simulink model "slow"  (R2019b)
settings: Solver=FixedStepDiscrete  StartTime=0.0  StopTime=25  FixedStep=Ts_ctrl  RelTol=1e-3
model workspace: external: MAT-File (data not in the file)
values from neighbouring files (symbols this model uses):
  CCR_max = 5250    [datasheet.m]
  delay_input = 0    [codegen_init.m]
  dpole_cut = exp(-w_cut*Ts_ctrl)    [codegen_init.m]
  encoder_res = 4096    [datasheet.m]
  g = 9.81    [datasheet.m]
  Jp = Jp_cm + mp*lp^2    (= 0.004290672)    [datasheet.m]
  Larm = 0.216    [datasheet.m]
  lp = 0.156    [datasheet.m]
  mp = 0.127    [datasheet.m]
  par_ctrl = Simulink.Parameter(par_ctrl)    [codegen_init.m]
  par_dn = Simulink.Parameter(par_dn)    [codegen_init.m]
  th_lim = 30/180*pi    (= 0.523598775598)    [codegen_init.m]
  Ts_ctrl = 5e-3    (= 0.005)    [codegen_init.m]
  volt_max = 6    [datasheet.m]
undefined symbols (not defined in the file or in its folder): state_board_init, state_pc_init
settings Model: OrderedModelArguments=off  Creator=Simone  LastModifiedBy=simone
settings OptimizationCC: DefaultParameterBehavior=Inlined  GainParamInheritBuiltInType=on  UseFloatMulNetSlope=on  UseSpecifiedMinMax=on  InlineInvariantSignals=on  PassReuseOutputArgsAs=Individual arguments  ZeroExternalMemoryAtStartup=off  ZeroInternalMemoryAtStartup=off  NoFixptDivByZeroProtection=on  EfficientFloat2IntCast=on  LifeSpan=1  OptimizeBlockOrder=speed  EfficientTunableParamExpr=on
settings DebuggingCC: SignalInfNanChecking=error  ParameterPrecisionLossMsg=error  ParameterTunabilityLossMsg=error
settings HardwareCC: ProdBitPerLong=64  ProdLongLongMode=on  ProdHWDeviceType=Intel->x86-64 (Linux 64)
settings SFSimCC: MATLABDynamicMemAlloc=off
settings RTWCC: SystemTargetFile=ert.tlc  GenCodeOnly=on  PackageGeneratedCodeAndArtifacts=on  TemplateMakefile=ert_default_tmf  GenerateReport=on  Toolchain=GNU gcc/g++ | gmake (64-bit Linux)  BuildConfiguration=Faster Runs  IncludeHyperlinkInReport=on  LaunchReport=on  GenerateTraceInfo=on  GenerateTraceReport=on  GenerateTraceReportSl=on  GenerateTraceReportSf=on  GenerateTraceReportEml=on  CheckMdlBeforeBuild=Error
settings CodeAppCC: ForceParamTrailComments=on  IgnoreCustomStorageClasses=off  OperatorAnnotations=on  SimulinkDataObjDesc=on  SFDataObjDesc=on  MATLABFcnDesc=on  InsertBlockDesc=on  StateflowObjectComments=on  MATLABSourceComments=on  EnableCustomComments=on  ReqsInCode=on
settings ERTTargetCC: TargetLangStandard=C99 (ISO)  UtilityFuncGeneration=Shared location  CombineSignalStateStructs=on  SuppressErrorStatus=on  SupportAbsoluteTime=off  SupportNonFinite=off  SupportComplex=off  InlinedParameterPlacement=NonHierarchical  ERTCustomFileTemplate=example_file_process.tlc

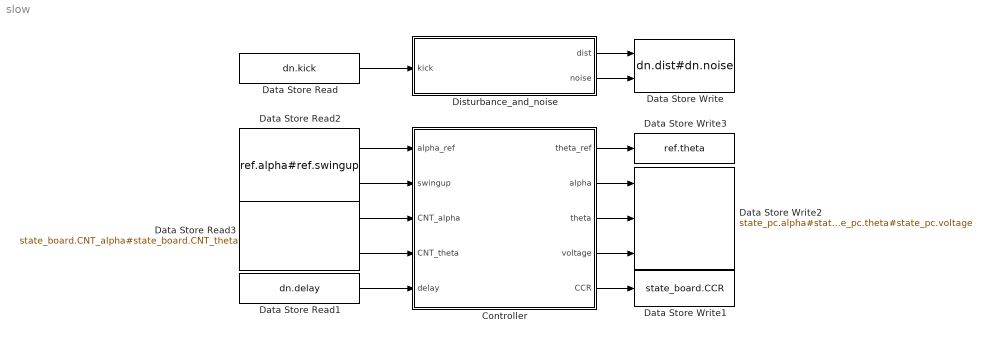
== system slow ==
  Controller : Subsystem  TreatAsAtomicUnit=on  RTWFcnName=controller  RTWFileName=controller
      settings: RTWSystemCode=Nonreusable function  RTWFcnNameOpts=User specified  RTWFileNameOpts=User specified  FunctionInterfaceSpec=Allow arguments
  Data Store Read : DataStoreRead  DataStoreName=dn  DataStoreElements=dn.kick
  Data Store Read1 : DataStoreRead  DataStoreName=dn  DataStoreElements=dn.delay
  Data Store Read2 : DataStoreRead  DataStoreName=ref  DataStoreElements=ref.alpha#ref.swingup
  Data Store Read3 : DataStoreRead  DataStoreName=state_board  DataStoreElements=state_board.CNT_alpha#state_board.CNT_theta
  Data Store Write : DataStoreWrite  DataStoreName=dn  DataStoreElements=dn.dist#dn.noise
  Data Store Write1 : DataStoreWrite  DataStoreName=state_board  DataStoreElements=state_board.CCR
  Data Store Write2 : DataStoreWrite  DataStoreName=state_pc  DataStoreElements=state_pc.alpha#state_pc.theta#state_pc.voltage
  Data Store Write3 : DataStoreWrite  DataStoreName=ref  DataStoreElements=ref.theta
  Disturbance_and_noise : Subsystem  TreatAsAtomicUnit=on  RTWFcnName=disturbance_and_noise  RTWFileName=disturbance_and_noise
      settings: RTWSystemCode=Nonreusable function  RTWFcnNameOpts=User specified  RTWFileNameOpts=User specified  FunctionInterfaceSpec=Allow arguments
  wires:
  Disturbance_and_noise/1(dist) -> Data Store Write/1
  Disturbance_and_noise/2(noise) -> Data Store Write/2
  Data Store Read/1 -> Disturbance_and_noise/1(kick)
  Controller/5(CCR) -> Data Store Write1/1
  Data Store Read2/2 -> Controller/2(swingup)
  Data Store Read2/1 -> Controller/1(alpha_ref)
  Data Store Read3/1 -> Controller/3(CNT_alpha)
  Data Store Read3/2 -> Controller/4(CNT_theta)
  Controller/4(voltage) -> Data Store Write2/3
  Controller/1(theta_ref) -> Data Store Write3/1
  Controller/3(theta) -> Data Store Write2/2
  Controller/2(alpha) -> Data Store Write2/1
  Data Store Read1/1 -> Controller/5(delay)

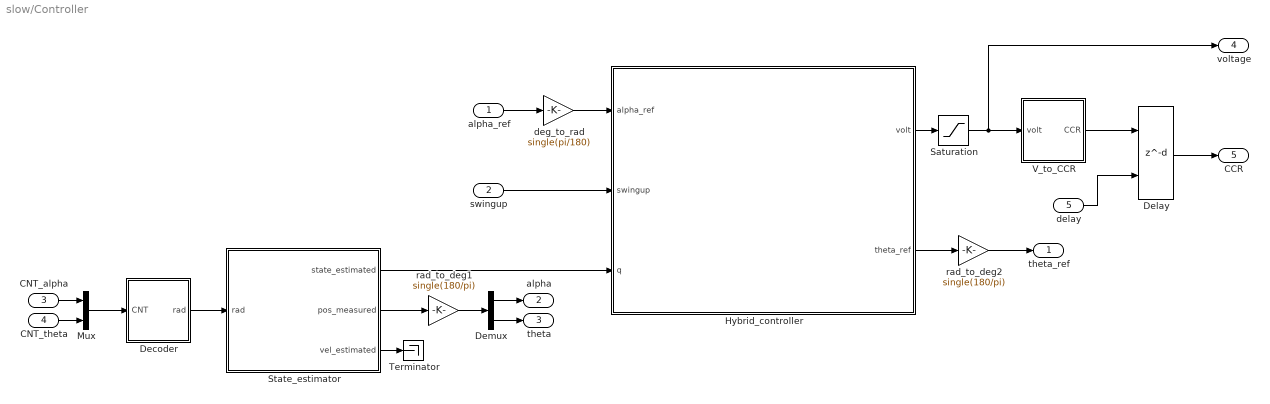
== system slow/Controller ==
  alpha_ref : Inport
  swingup : Inport  Port=2
  CNT_alpha : Inport  Port=3
  CNT_theta : Inport  Port=4
  delay : Inport  Port=5
  Decoder : Subsystem
  Delay : Delay  DelayLengthSource=Input port  DelayLength=delay_input  DelayLengthUpperLimit=255  InitialCondition=state_board_init.CCR
      settings: InputPortMap=u0,p1
  Demux : Demux  Outputs=2
  Hybrid_controller : Stateflow chart  BlockKeywords=__PRM__SERIALIZED__DATA__:Stateflow Chart,Stateflow Diagram  TreatAsAtomicUnit=on
  Mux : Mux  Inputs=2
  Saturation : Saturate  UpperLimit=volt_max  LowerLimit=-volt_max
  State_estimator : Subsystem
  Terminator : Terminator
  V_to_CCR : Subsystem
  deg_to_rad : Gain  Gain=single(pi/180)
  rad_to_deg1 : Gain  Gain=single(180/pi)
  rad_to_deg2 : Gain  Gain=single(180/pi)
  theta_ref : Outport
  alpha : Outport  Port=2
  theta : Outport  Port=3
  voltage : Outport  Port=4
  CCR : Outport  Port=5
  wires:
  Saturation/1 -> voltage/1, V_to_CCR/1(volt)
  Delay/1 -> CCR/1
  rad_to_deg2/1 -> theta_ref/1
  Demux/1 -> alpha/1
  Demux/2 -> theta/1
  State_estimator/1(state_estimated) -> Hybrid_controller/3(q)
  State_estimator/3(vel_estimated) -> Terminator/1
  deg_to_rad/1 -> Hybrid_controller/1(alpha_ref)
  delay/1 -> Delay/2
  CNT_theta/1 -> Mux/2
  Mux/1 -> Decoder/1(CNT)
  rad_to_deg1/1 -> Demux/1
  Hybrid_controller/2(theta_ref) -> rad_to_deg2/1
  swingup/1 -> Hybrid_controller/2(swingup)
  alpha_ref/1 -> deg_to_rad/1
  Decoder/1(rad) -> State_estimator/1(rad)
  CNT_alpha/1 -> Mux/1
  State_estimator/2(pos_measured) -> rad_to_deg1/1
  V_to_CCR/1(CCR) -> Delay/1
  Hybrid_controller/1(volt) -> Saturation/1

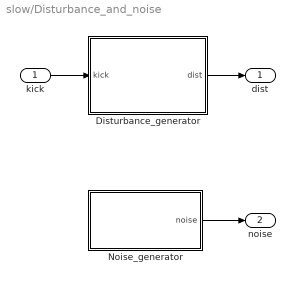
== system slow/Disturbance_and_noise ==
  kick : Inport
  Disturbance_generator : Stateflow chart  BlockKeywords=__PRM__SERIALIZED__DATA__:Stateflow Chart,Stateflow Diagram  TreatAsAtomicUnit=on
  Noise_generator : Subsystem
  dist : Outport
  noise : Outport  Port=2
  wires:
  Disturbance_generator/1(dist) -> dist/1
  Noise_generator/1(noise) -> noise/1
  kick/1 -> Disturbance_generator/1(kick)

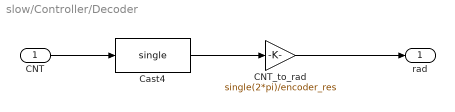
== system slow/Controller/Decoder ==
  CNT : Inport
  CNT_to_rad : Gain  Gain=single(2*pi)/encoder_res
  Cast4 : DataTypeConversion  OutDataTypeStr=single
  rad : Outport
  wires:
  Cast4/1 -> CNT_to_rad/1
  CNT/1 -> Cast4/1
  CNT_to_rad/1 -> rad/1

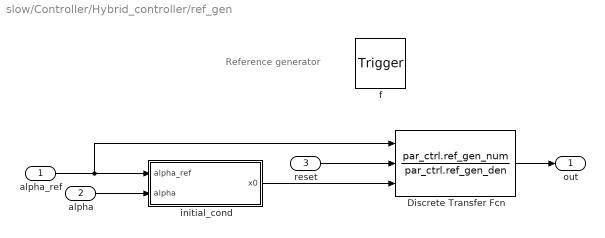
== system slow/Controller/Hybrid_controller/ref_gen ==
  note: Reference generator
  alpha_ref : Inport  OutDataTypeStr=single  PortDimensions=1
  alpha : Inport  Port=2  OutDataTypeStr=single  PortDimensions=1
  reset : Inport  Port=3  OutDataTypeStr=int8  PortDimensions=1
  f : TriggerPort  TriggerType=function-call  VariantControl=(inherit)
      settings: CopyFcn=Stateflow.SLINSF.SimulinkMan.removeBlockPreDeleteFcn  PreDeleteFcn=Stateflow.SLINSF.SimulinkMan.unsafePredeleteFcn
  Discrete Transfer Fcn : DiscreteTransferFcn  Numerator=par_ctrl.ref_gen_num  Denominator=par_ctrl.ref_gen_den  InitialStatesSource=Input port  ExternalReset=Falling
      settings: InputPortMap=u0,r7,p5
  initial_cond : MATLAB Function
  out : Outport  OutDataTypeStr=single
  wires:
  alpha_ref/1 -> Discrete Transfer Fcn/1, initial_cond/1(alpha_ref)
  alpha/1 -> initial_cond/2(alpha)
  reset/1 -> Discrete Transfer Fcn/2
  Discrete Transfer Fcn/1 -> out/1
  initial_cond/1(x0) -> Discrete Transfer Fcn/3

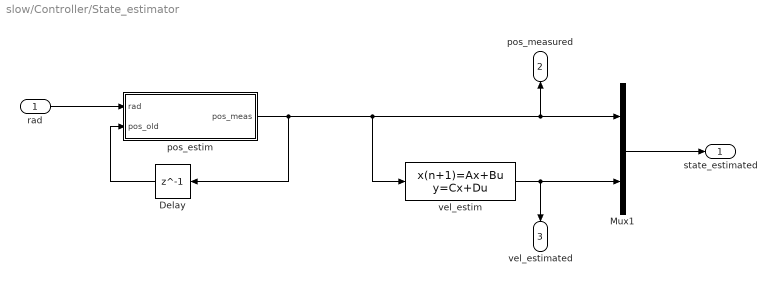
== system slow/Controller/State_estimator ==
  rad : Inport
  Delay : Delay  DelayLength=1  InitialCondition=[state_pc_init.alpha;state_pc_init.theta]
  Mux1 : Mux  Inputs=2
  pos_estim : MATLAB Function
  vel_estim : DiscreteStateSpace  A=dpole_cut*eye(2)  B=eye(2)  C=-1/single(Ts_ctrl)*(1-dpole_cut)^2*eye(2)  D=(1-dpole_cut)/single(Ts_ctrl)*eye(2)  InitialCondition=1/(1-dpole_cut)*eye(2)*[state_pc_init.alpha;state_pc_init.theta]  SampleTime=Ts_ctrl
  state_estimated : Outport
  pos_measured : Outport  Port=2
  vel_estimated : Outport  Port=3
  wires:
  vel_estim/1 -> Mux1/2, vel_estimated/1
  Delay/1 -> pos_estim/2(pos_old)
  rad/1 -> pos_estim/1(rad)
  Mux1/1 -> state_estimated/1
  pos_estim/1(pos_meas) -> Mux1/1, pos_measured/1, vel_estim/1, Delay/1

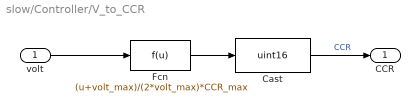
== system slow/Controller/V_to_CCR ==
  volt : Inport
  Cast : DataTypeConversion  OutDataTypeStr=uint16  RndMeth=Round
  Fcn : Fcn  Expr=(u+volt_max)/(2*volt_max)*CCR_max
  CCR : Outport
  wires:
  Fcn/1 -> Cast/1
  Cast/1 -> CCR/1  "CCR"
  volt/1 -> Fcn/1

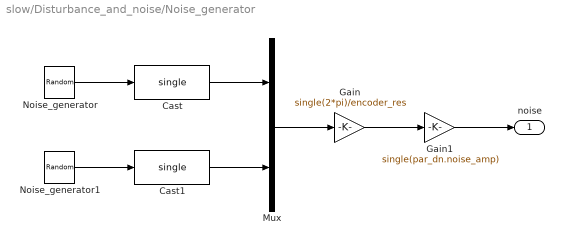
== system slow/Disturbance_and_noise/Noise_generator ==
  Cast : DataTypeConversion  OutDataTypeStr=single
  Cast1 : DataTypeConversion  OutDataTypeStr=single
  Gain : Gain  Gain=single(2*pi)/encoder_res
  Gain1 : Gain  Gain=single(par_dn.noise_amp)
  Mux : Mux  Inputs=2
  Noise_generator : UniformRandomNumber  Seed=2342  SampleTime=Ts_ctrl
  Noise_generator1 : UniformRandomNumber  Seed=1558  SampleTime=Ts_ctrl
  noise : Outport
  wires:
  Mux/1 -> Gain/1
  Gain1/1 -> noise/1
  Gain/1 -> Gain1/1
  Noise_generator/1 -> Cast/1
  Noise_generator1/1 -> Cast1/1
  Cast/1 -> Mux/1
  Cast1/1 -> Mux/2

== matlab function slow/Controller/State_estimator/pos_estim ==
  data: rad input single; pos_old input single; pos_meas output single
function pos_meas = pos_estim(rad,pos_old)

sect = @(th)mod(int8(floor(th/single(pi/2))),int8(4));

pos_meas = floor(pos_old/single(2*pi))*single(2*pi) +...
           mod(rad,single(2*pi));

for k=1:2
    if sect(pos_old(k)) == int8(3) && sect(rad(k)) == int8(0)
        pos_meas(k) = pos_meas(k) + single(2*pi);
    elseif sect(pos_old(k)) == int8(0) && sect(rad(k)) == int8(3)
        pos_meas(k) = pos_meas(k) - single(2*pi);
    end
end

== stateflow chart slow/Controller/Hybrid_controller ==
  settings: sampleTime=Ts_ctrl
  state PD_controller_up
    entry:
    ref_gen(alpha_ref,q(1),int8(1));
    theta_ref = round(q(2)/single(2*pi))*single(2*pi);
    entry, during:
    K = [par_ctrl.up_kp_alpha,...
    par_ctrl.up_kp_theta,...
    par_ctrl.up_kd_alpha,...
    par_ctrl.up_kd_theta];
    contr_pd;
  state Sliding_mode_controller
    during:
    theta_ref = round(q(2)/single(2*pi))*single(2*pi);
    state Idle
      during:
      volt = 0;
    state Swing_up
      entry, during:
      contr_su;
    Swing_up -> Idle : [energy(q) >= 0]
    (default) -> Idle
    Idle -> Swing_up : [energy(q) < 0]
  state PD_controller_down
    entry:
    ref_gen(alpha_ref,q(1),int8(1));
    entry, during:
    theta_ref = (round(q(2)/single(2*pi)+0.5)-0.5)*single(2*pi);
    K = [par_ctrl.down_kp_alpha,...
    single(0),...
    par_ctrl.down_kd_alpha,...
    single(0)];
    contr_pd;
  state out = ref_gen(alpha_ref,alpha,reset) [function]
  Sliding_mode_controller -> PD_controller_up [order 1] : [swingup == 1 &&...
      | abs(q(2)-round(q(2)/(2*pi))*2*pi) <= th_lim]
  PD_controller_up -> Sliding_mode_controller : [swingup == 0 ||...
      | abs(q(2)-round(q(2)/(2*pi))*2*pi) > th_lim]
  (default) -> Sliding_mode_controller
  PD_controller_down -> Sliding_mode_controller : [swingup == 1]
  Sliding_mode_controller -> PD_controller_down [order 2] : [swingup == 0]
  data: volt_max parameter; state function_input single; Jp parameter; Larm parameter; g parameter; lp parameter; mp parameter; ME function_output single; alpha_ref function_input single size=1; out function_output single; alpha function_input single size=1; reset function_input int8 size=1; alpha_ref input single; volt output single =single(0); swingup input uint8; q input single; th_lim parameter; K local single; par_ctrl parameter; theta_ref output single =single(pi)
  function contr_su:
    | % Swing-up controller
    | 
    | function contr_su
    | 
    | th = q(2);
    | th_d = q(4);
    | 
    | if th_d*cos(th) == 0
    |     sgn = sign(th);
    | else
    |     sgn = sign(th_d*cos(th));
    | end
    | 
    | volt = -volt_max*sgn;
  function contr_pd:
    | % PD controller with reference generator
    | 
    | function contr_pd
    | 
    | q_ref = [ref_gen(alpha_ref,q(1),int8(0)); theta_ref; 0; 0];
    | error = q_ref - q;
    | volt = K * error;
  function ME = energy(state):
    | % Mechanical energy calculation (kinetic + potential)
    | 
    | function ME = energy(state)
    | 
    | th = state(2);
    | al_d = state(3);
    | th_d = state(4);
    | 
    | ME = (Jp*al_d^2)/2 + (Jp*th_d^2)/2 + (Larm^2*al_d^2*mp)/2 - g*lp*mp - (Jp*al_d^2*cos(th)^2)/2 + g*lp*mp*cos(th) + Larm*al_d*lp*mp*th_d*cos(th);

== stateflow chart slow/Disturbance_and_noise/Disturbance_generator ==
  settings: sampleTime=Ts_ctrl
  state Reset
    entry:
    dist = 0;
  state Off
  state On
    entry:
    dist = par_dn.dist_amp;
  (default) -> Reset
  On -> Reset : after(10,tick)
  Reset -> Off : [kick == 0]
  Off -> On : [kick == 1]
  data: kick input uint8; dist output single =single(0); par_dn parameter

== matlab function slow/Controller/Hybrid_controller/ref_gen/initial_cond ==
  data: alpha_ref input; x0 output; alpha input; par_ctrl parameter
function x0 = initial_cond(alpha_ref, alpha, par_ctrl)

x0 = 1/par_ctrl.dpole_ref*(alpha/(1-par_ctrl.dpole_ref)-alpha_ref);
